simulink model "MIC_Mdl_IdentFilter"  (R2025b)
settings: Solver=ode15s  StartTime=0.0  StopTime=10  FixedStep=0.001  RelTol=1e-6  AbsTol=1e-6  EnableMultiTasking=on
values from neighbouring files (symbols this model uses):
  Alpha1Flag = 0    [Compare.m]
  IdentTs = SimuRunInfo.IdentTs    [Compare.m]
undefined symbols (not defined in the file or in its folder): Difwn, DifZeta, Identwn, IdentZeta
settings Model: Creator=wzj  LastModifiedBy=ASUS
settings SolverCC: AlgebraicLoopSolver=TrustRegion
settings DataIOCC: LimitDataPoints=on  SaveFormat=Array  ReturnWorkspaceOutputs=off
settings OptimizationCC: ReuseModelBlockBuffer=off  LifeSpan=inf
settings DebuggingCC: UnderspecifiedInitializationDetection=Classic  MergeDetectMultiDrivingBlocksExec=none  SolverPrmCheckMsg=warning  UnconnectedInputMsg=warning  UnconnectedOutputMsg=warning  UnconnectedLineMsg=warning  StateNameClashWarn=warning  SFUnexpectedBacktrackingDiag=warning  SFNoUnconditionalDefaultTransitionDiag=warning  SFExecutionAtInitializationDiag=none  ArithmeticOperatorsInVariantConditions=warning
settings HardwareCC: ProdBitPerPointer=32.0  ProdBitPerSizeT=32.0  ProdBitPerPtrDiffT=32.0  ProdLargestAtomicFloat=None  ProdIntDivRoundTo=Undefined  ProdEndianess=Unspecified  ProdWordSize=32.0  ProdHWDeviceType=32-bit Generic
settings ModelReferenceCC: EnableRefExpFcnMdlSchedulingChecks=on  PropagateSignalLabelsOutOfModel=off
settings SFSimCC: SimUseLocalCustomCode=off  CustomCodeUndefinedFunction=UseInterfaceOnly
settings RTWCC: RTWUseLocalCustomCode=off  GPUComputeCapability=3.5
settings CodeAppCC: StateflowObjectComments=on
settings GRTTargetCC: TargetLangStandard=C89/C90 (ANSI)
settings ConfigComp: CovMetricSettings=dw  CovSaveCumulativeToWorkspaceVar=on  CovSaveSingleToWorkspaceVar=on  CovExternalEMLEnable=off

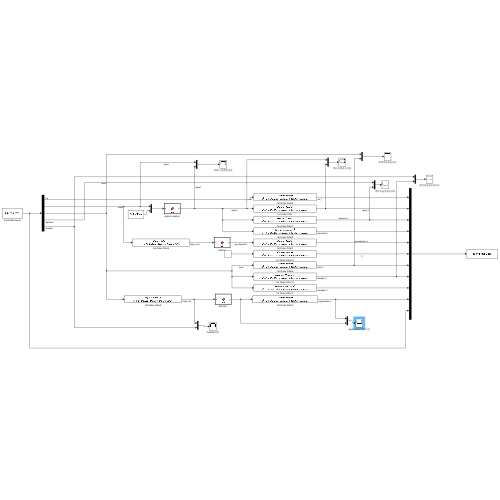
[thumbnail: Simulink's stored preview of the top-level diagram]
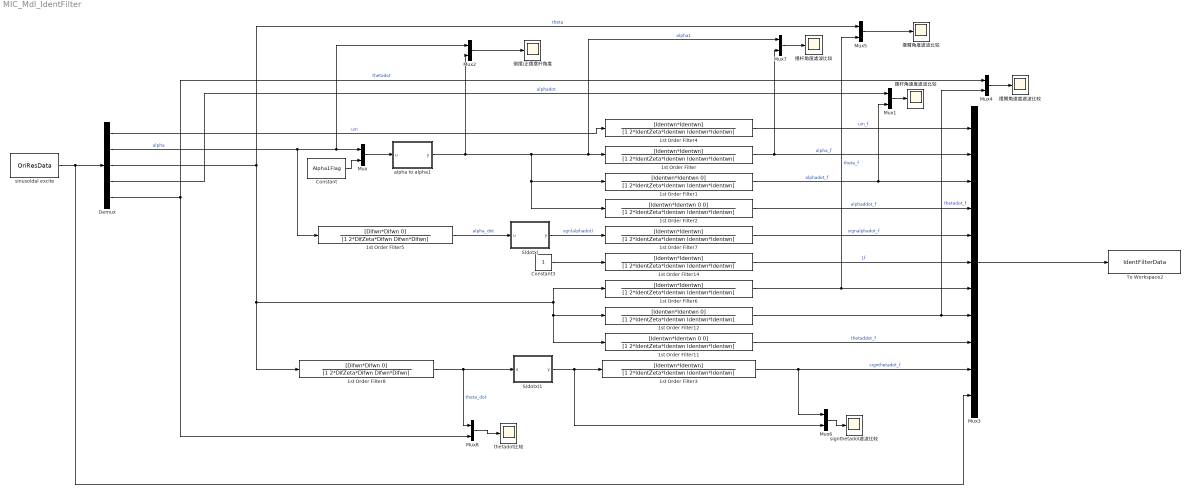
== system MIC_Mdl_IdentFilter ==
  1st Order Filter{,3..4,6..7,14} (6 alike) : TransferFcn  Numerator=[Identwn*Identwn]  Denominator=[1 2*IdentZeta*Identwn Identwn*Identwn]
  1st Order Filter1 : TransferFcn  Numerator=[Identwn*Identwn 0]  Denominator=[1 2*IdentZeta*Identwn Identwn*Identwn]
  1st Order Filter11 : TransferFcn  Numerator=[Identwn*Identwn 0 0]  Denominator=[1 2*IdentZeta*Identwn Identwn*Identwn]
  1st Order Filter12 : TransferFcn  Numerator=[Identwn*Identwn 0]  Denominator=[1 2*IdentZeta*Identwn Identwn*Identwn]
  1st Order Filter2 : TransferFcn  Numerator=[Identwn*Identwn 0 0]  Denominator=[1 2*IdentZeta*Identwn Identwn*Identwn]
  1st Order Filter5 : TransferFcn  Numerator=[Difwn*Difwn 0]  Denominator=[1 2*DifZeta*Difwn Difwn*Difwn]
  1st Order Filter8 : TransferFcn  Numerator=[Difwn*Difwn 0]  Denominator=[1 2*DifZeta*Difwn Difwn*Difwn]
  Constant : Constant  Value=Alpha1Flag
  Constant3 : Constant
  Demux : Demux  Outputs=5
  Mux{,1..2,4..8} (8 alike) : Mux  Inputs=2
  Mux3 : Mux  Inputs=11
  S(dotx) : MATLAB Function  TreatAsAtomicUnit=on
  S(dotx)1 : MATLAB Function  TreatAsAtomicUnit=on
  To Workspace2 : ToWorkspace  VariableName=IdentFilterData  SaveFormat=Structure With Time  SampleTime=IdentTs
  alpha to alpha1 : MATLAB Function  TreatAsAtomicUnit=on
  signthetadot滤波比较 : Scope
      settings: ActiveDisplayYMinimum=-1.25584  ActiveDisplayYMaximum=1.30254  DataLoggingVariableName=ScopeData10
  sinusoidal excite : FromWorkspace  VariableName=OriResData  SampleTime=IdentTs
  thetadot比较 : Scope
      settings: ActiveDisplayYMinimum=-1  ActiveDisplayYMaximum=1  DataLoggingVariableName=ScopeData30
  倒摆/正摆摆杆角度 : Scope
      settings: ActiveDisplayYMinimum=-1  ActiveDisplayYMaximum=1  DataLoggingVariableName=ScopeData2
  摆杆角度滤波比较 : Scope
      settings: ActiveDisplayYMinimum=-33.36263  ActiveDisplayYMaximum=29.9758  DataLoggingVariableName=ScopeData20
  摆杆角速度滤波比较 : Scope
      settings: ActiveDisplayYMinimum=-178.80726  ActiveDisplayYMaximum=198.03876
  摆臂角度滤波比较 : Scope
      settings: ActiveDisplayYMinimum=-4.45773  ActiveDisplayYMaximum=39.62489  DataLoggingVariableName=ScopeData5
  摆臂角速度滤波比较 : Scope
      settings: ActiveDisplayYMinimum=-109.24194  ActiveDisplayYMaximum=106.42555  DataLoggingVariableName=ScopeData4
  wires:
  1st Order Filter6/1 -> Mux3/7, Mux5/2  "theta_f"
  Demux/3 -> Mux5/1, 1st Order Filter11/1, 1st Order Filter12/1, 1st Order Filter6/1, 1st Order Filter8/1  "theta"
  alpha to alpha1/1(y) -> Mux2/2, 1st Order Filter2/1, 1st Order Filter1/1, Mux7/1, 1st Order Filter/1  "alpha1"
  Mux4/1 -> 摆臂角速度滤波比较/1
  Mux2/1 -> 倒摆/正摆摆杆角度/1
  Mux/1 -> alpha to alpha1/1(u)
  1st Order Filter4/1 -> Mux3/1  "uin_f"
  1st Order Filter3/1 -> Mux6/1, Mux3/10  "signthetadot_f"
  1st Order Filter12/1 -> Mux4/2, Mux3/8  "thetadot_f"
  Demux/1 -> 1st Order Filter4/1  "uin"
  1st Order Filter1/1 -> Mux1/2, Mux3/3  "alphadot_f"
  1st Order Filter14/1 -> Mux3/6  "1f"
  S(dotx)1/1(y) -> Mux6/2, 1st Order Filter3/1
  Constant3/1 -> 1st Order Filter14/1
  Demux/2 -> Mux2/1, Mux/1, 1st Order Filter5/1  "alpha"
  1st Order Filter11/1 -> Mux3/9  "thetaddot_f"
  S(dotx)/1(y) -> 1st Order Filter7/1  "sgn(alphadot)"
  Mux5/1 -> 摆臂角度滤波比较/1
  1st Order Filter2/1 -> Mux3/4  "alphaddot_f"
  1st Order Filter/1 -> Mux7/2, Mux3/2  "alpha_f"
  1st Order Filter7/1 -> Mux3/5  "signalphadot_f"
  Mux3/1 -> To Workspace2/1
  1st Order Filter5/1 -> S(dotx)/1(u)  "alpha_dot"
  1st Order Filter8/1 -> Mux8/1, S(dotx)1/1(u)  "theta_dot"
  Mux1/1 -> 摆杆角速度滤波比较/1
  Mux7/1 -> 摆杆角度滤波比较/1
  sinusoidal excite/1 -> Mux3/11, Demux/1
  Constant/1 -> Mux/2
  Demux/5 -> Mux8/2, Mux4/1  "thetadot"
  Demux/4 -> Mux1/1  "alphadot"
  Mux6/1 -> signthetadot滤波比较/1
  Mux8/1 -> thetadot比较/1

== matlab function MIC_Mdl_IdentFilter/S(dotx)1 ==
  data: u input; y output
function y = fcn(u)

%y = 2/pi*atan(900*u);
signcoef=1e3;
y = tanh(signcoef*u);

== matlab function MIC_Mdl_IdentFilter/alpha to alpha1 ==
  data: u input; y output
function y = fcn(u)
 alpha = u(1); %rad
 flag1 = u(2);
if(flag1 >0.5) %flag ==1: alpha1=alpha-pi; flag ==0: alpha1 =alpha
  alpha1 = alpha - 180;
else
    alpha1 = alpha;
end
y = alpha1;

== matlab function MIC_Mdl_IdentFilter/S(dotx) ==
  data: u input; y output
function y = fcn(u)

%y = 2/pi*atan(900*u);
signcoef=1e3;
y = tanh(signcoef*u);
